simulink model "am"  (Simulink 7.6)
settings: Solver=ode45  StartTime=0.0  StopTime=10.0  RelTol=1e-3
settings Model: Creator=Felipe Bandeira  LastModifiedBy=Felipe Bandeira

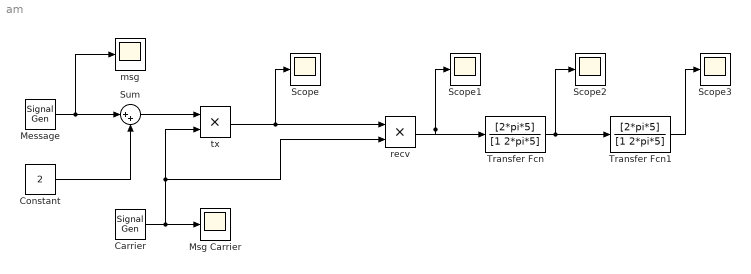
== system am ==
  Carrier : SignalGenerator  Frequency=20
  Constant : Constant  Value=2
  Message : SignalGenerator
  Msg Carrier : Scope
      settings: SaveName=ScopeData2
  Scope{,1..3} (4 alike) : Scope
      Scope1 settings: SaveName=ScopeData3
      Scope2 settings: SaveName=ScopeData4
      Scope3 settings: SaveName=ScopeData5
  Sum : Sum  Inputs=|++
  Transfer Fcn : TransferFcn  Numerator=[2*pi*5]  Denominator=[1 2*pi*5]
  Transfer Fcn1 : TransferFcn  Numerator=[2*pi*5]  Denominator=[1 2*pi*5]
  msg : Scope
  recv : Product  RndMeth=Zero
  tx : Product  SampleTime=0.001  RndMeth=Zero
  wires:
  Message/1 -> Sum/1, msg/1
  Constant/1 -> Sum/2
  Sum/1 -> tx/1
  Carrier/1 -> Msg Carrier/1, tx/2, recv/2
  tx/1 -> Scope/1, recv/1
  recv/1 -> Scope1/1, Transfer Fcn/1
  Transfer Fcn/1 -> Scope2/1, Transfer Fcn1/1
  Transfer Fcn1/1 -> Scope3/1
